simulink model "Filter"  (R2020b)
settings: Solver=VariableStepAuto  StartTime=0.0  StopTime=10.0  RelTol=1e-3
settings Model: Creator=Shubham  LastModifiedBy=Shubham

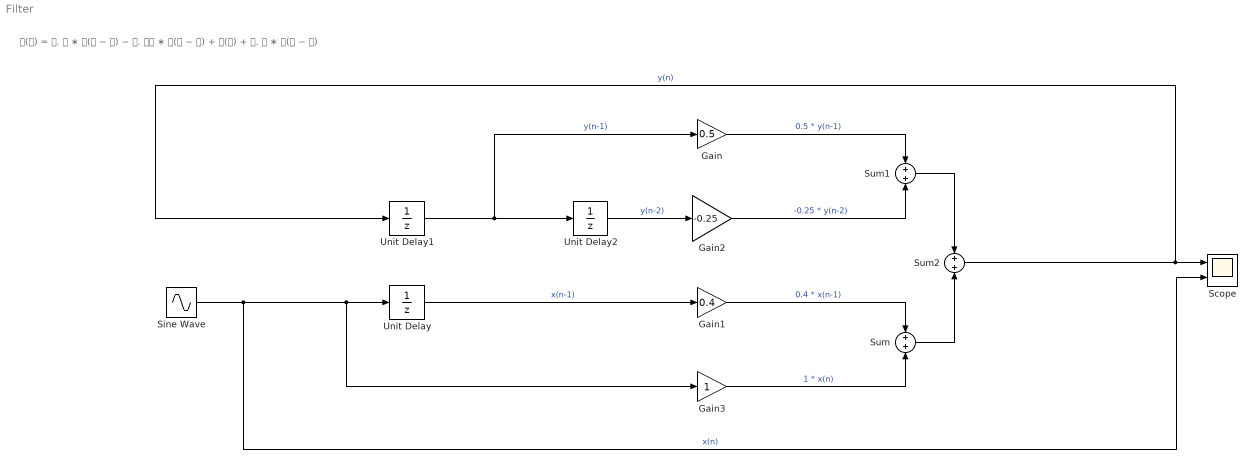
== system Filter ==
  note: 𝐲(𝐧) = 𝟎. 𝟓 ∗ 𝐲(𝐧 − 𝟏) − 𝟎. 𝟐𝟓 ∗ 𝐲(𝐧 − 𝟐) + 𝐱(𝐧) + 𝟎. 𝟒 ∗ 𝐱(𝐧 − 𝟏)
  Gain : Gain  Gain=0.5
  Gain1 : Gain  Gain=0.4
  Gain2 : Gain  Gain=-0.25
  Gain3 : Gain
  Scope : Scope  NumInputPorts=2
  Sine Wave : Sin  SampleTime=0
  Sum : Sum
  Sum1 : Sum
  Sum2 : Sum
  Unit Delay : UnitDelay  SampleTime=-1  HasFrameUpgradeWarning=on
  Unit Delay1 : UnitDelay  SampleTime=-1  HasFrameUpgradeWarning=on
  Unit Delay2 : UnitDelay  SampleTime=-1  HasFrameUpgradeWarning=on
  wires:
  Sine Wave/1 -> Scope/2, Gain3/1, Unit Delay/1  "x(n)"
  Unit Delay/1 -> Gain1/1  "x(n-1)"
  Unit Delay1/1 -> Gain/1, Unit Delay2/1  "y(n-1)"
  Unit Delay2/1 -> Gain2/1  "y(n-2)"
  Gain/1 -> Sum1/1  "0.5 * y(n-1)"
  Gain2/1 -> Sum1/2  "-0.25 * y(n-2)"
  Gain1/1 -> Sum/1  "0.4 * x(n-1)"
  Gain3/1 -> Sum/2  "1 * x(n)"
  Sum2/1 -> Unit Delay1/1, Scope/1  "y(n)"
  Sum1/1 -> Sum2/1
  Sum/1 -> Sum2/2
